simulink model "workingAUTOdec8"  (R2023b)
settings: Solver=FixedStepAuto  StartTime=0.0  StopTime=inf  RelTol=1e-3  EnableMultiTasking=on
libraries: vexarmcortexlib x17, vexcommonlib x4
settings Model: Creator=carol  LastModifiedBy=carol
settings SolverCC: AutoInsertRateTranBlk=on
settings DataIOCC: LimitDataPoints=on  SignalLoggingSaveFormat=ModelDataLogs  ReturnWorkspaceOutputs=off
settings OptimizationCC: ExpressionDepthLimit=2147483647  LifeSpan=Inf  MaxStackSize=64  EfficientTunableParamExpr=on
settings DebuggingCC: MergeDetectMultiDrivingBlocksExec=none  InheritedTsInSrcMsg=none  MultiTaskCondExecSysMsg=none  FcnCallInpInsideContextMsg=warning  StateNameClashWarn=warning  SFUnexpectedBacktrackingDiag=warning  SFNoUnconditionalDefaultTransitionDiag=warning  SFExecutionAtInitializationDiag=none  ArithmeticOperatorsInVariantConditions=warning
settings HardwareCC: ProdBitPerPointer=32  ProdBitPerSizeT=32  ProdBitPerPtrDiffT=32  ProdLargestAtomicInteger=Long  ProdLargestAtomicFloat=Double  ProdIntDivRoundTo=Undefined  ProdWordSize=32  ProdHWDeviceType=ARM Compatible->ARM Cortex
settings ModelReferenceCC: EnableRefExpFcnMdlSchedulingChecks=on  PropagateSignalLabelsOutOfModel=off
settings SFSimCC: MATLABDynamicMemAlloc=off  CustomCodeUndefinedFunction=UseInterfaceOnly
settings RTWCC: Description=Embedded Coder  SystemTargetFile=ert.tlc  HardwareBoard=ARM Cortex-based VEX Microcontroller  TemplateMakefile=ert_default_tmf  Toolchain=GNU Tools for VEX ARM Cortex
settings CodeAppCC: IgnoreCustomStorageClasses=off  CustomSymbolStrType=$N$R$M  StateflowObjectComments=on  InternalIdentifier=Classic
settings ERTTargetCC: CodeReplacementLibrary=GCC ARM Cortex-M3  MultiwordLength=2048  ConvertIfToSwitch=off  SuppressUnreachableDefaultCases=off

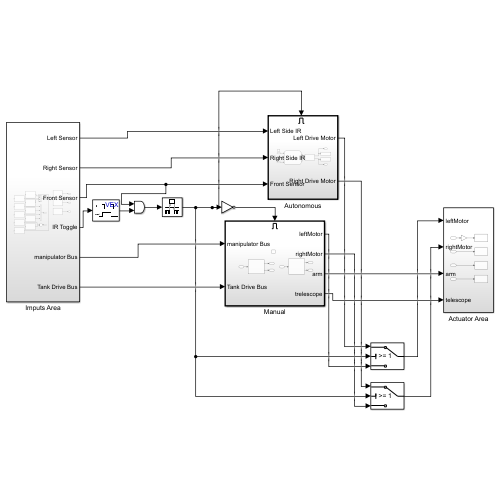
[thumbnail: Simulink's stored preview of the top-level diagram]
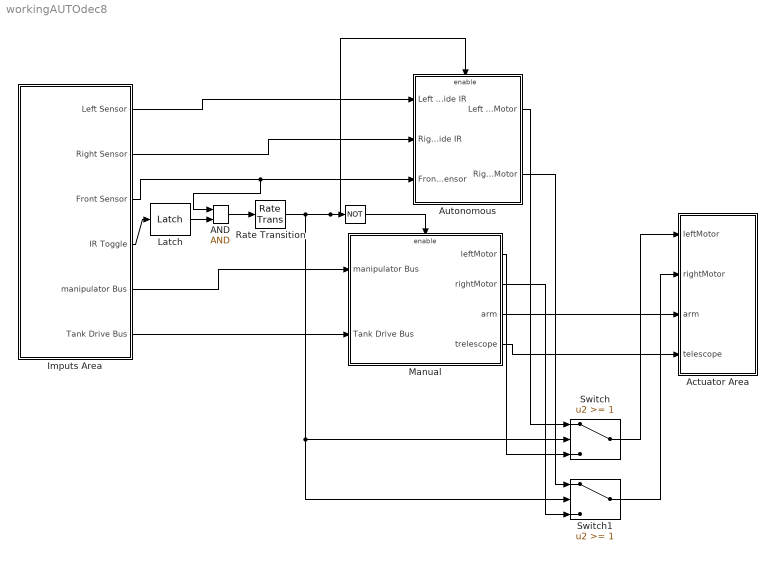
== system workingAUTOdec8 ==
  " " : Logic  Operator=NOT  IconShape=distinctive  AllPortsSameDT=off  OutDataTypeStr=boolean
  AND : Logic  IconShape=distinctive  AllPortsSameDT=off  OutDataTypeStr=boolean
  Actuator Area : Subsystem
  Autonomous : Subsystem  TreatAsAtomicUnit=on
  Imputs Area : Subsystem
  Latch : vexcommonlib/Latch  output0=off  BlockPlatform=vexarmcortex
  Manual : Subsystem  TreatAsAtomicUnit=on
  Rate Transition : RateTransition
  Switch : Switch  Threshold=1  SaturateOnIntegerOverflow=off  InputSameDT=off
  Switch1 : Switch  Threshold=1  SaturateOnIntegerOverflow=off  InputSameDT=off
  wires:
  Manual/3(arm) -> Actuator Area/3(arm)
  Manual/4(trelescope) -> Actuator Area/4(telescope)
  Switch1/1 -> Actuator Area/2(rightMotor)
  Switch/1 -> Actuator Area/1(leftMotor)
  Imputs Area/2(Right Sensor) -> Autonomous/2(Right Side IR)
  Imputs Area/3(Front Sensor) -> Autonomous/3(Front Sensor), AND/1
  Imputs Area/1(Left Sensor) -> Autonomous/1(Left Side IR)
  Imputs Area/5(manipulator Bus) -> Manual/1(manipulator Bus)
  Imputs Area/6(Tank Drive Bus) -> Manual/2(Tank Drive Bus)
  AND/1 -> Rate Transition/1
  Imputs Area/4(IR Toggle) -> Latch/1
  Latch/1 -> AND/2
  " "/1 -> Manual/Enable
  Autonomous/1(Left Drive Motor) -> Switch/1
  Manual/1(leftMotor) -> Switch/3
  Autonomous/2(Right Drive Motor) -> Switch1/1
  Manual/2(rightMotor) -> Switch1/3
  Rate Transition/1 -> Switch1/2, Switch/2, Autonomous/Enable, " "/1

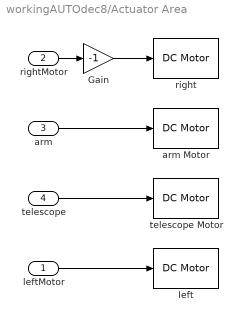
== system workingAUTOdec8/Actuator Area ==
  leftMotor : Inport
  rightMotor : Inport  Port=2
  arm : Inport  Port=3
  telescope : Inport  Port=4
  Gain : Gain  Gain=-1
  arm Motor : vexarmcortexlib/Actuators/DC Motor  motor=6  scaleFactor=1/13.5  SimulationOut=off
  left : vexarmcortexlib/Actuators/DC Motor  motor=9  scaleFactor=1/13.5  SimulationOut=off
  right : vexarmcortexlib/Actuators/DC Motor  motor=2  scaleFactor=1/13.5  SimulationOut=off
  telescope Motor : vexarmcortexlib/Actuators/DC Motor  motor=5  scaleFactor=1/13.5  SimulationOut=off
  wires:
  leftMotor/1 -> left/1
  arm/1 -> arm Motor/1
  rightMotor/1 -> Gain/1
  telescope/1 -> telescope Motor/1
  Gain/1 -> right/1

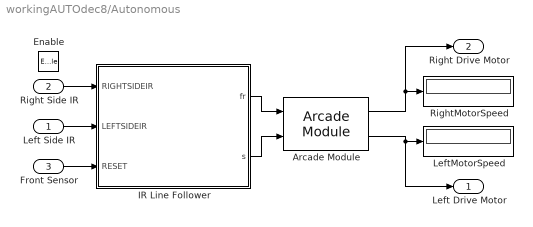
== system workingAUTOdec8/Autonomous ==
  Left Side IR : Inport
  Right Side IR : Inport  Port=2
  Front Sensor : Inport  Port=3
  Enable : EnablePort  StatesWhenEnabling=reset
  Arcade Module : vexcommonlib/Arcade Module  BlockPlatform=vexarmcortex
  IR Line Follower : Stateflow chart  TreatAsAtomicUnit=on
  LeftMotorSpeed : Display
  RightMotorSpeed : Display
  Left Drive Motor : Outport
  Right Drive Motor : Outport  Port=2
  wires:
  Arcade Module/2 -> LeftMotorSpeed/1, Left Drive Motor/1
  Arcade Module/1 -> Right Drive Motor/1, RightMotorSpeed/1
  Front Sensor/1 -> IR Line Follower/3(RESET)
  IR Line Follower/1(fr) -> Arcade Module/1
  IR Line Follower/2(s) -> Arcade Module/2
  Right Side IR/1 -> IR Line Follower/1(RIGHTSIDEIR)
  Left Side IR/1 -> IR Line Follower/2(LEFTSIDEIR)

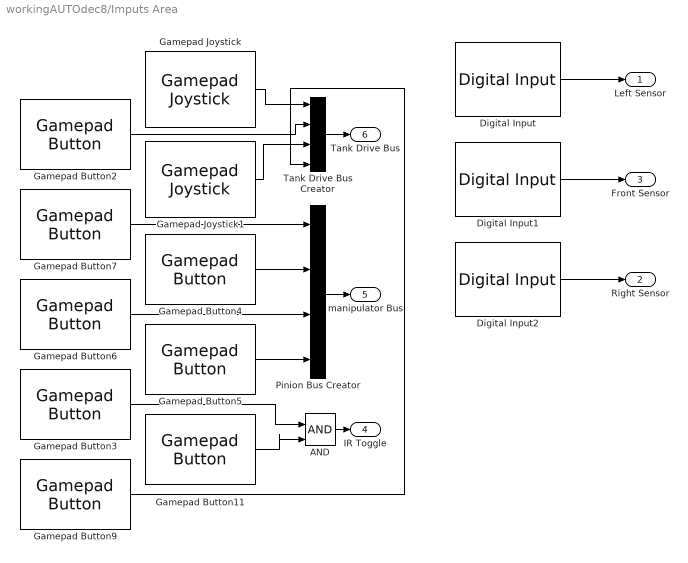
== system workingAUTOdec8/Imputs Area ==
  AND : Logic  IconShape=distinctive  AllPortsSameDT=off  OutDataTypeStr=boolean
  Digital Input : vexarmcortexlib/Sensors/Digital Input  inChan=10  SimulationIn=off  SampleTime=0.002
  Digital Input1 : vexarmcortexlib/Sensors/Digital Input  inChan=11  SimulationIn=off  SampleTime=0.002
  Digital Input2 : vexarmcortexlib/Sensors/Digital Input  inChan=12  SimulationIn=off  SampleTime=0.002
  Gamepad Button11 : vexarmcortexlib/Gamepad/Gamepad Button  joystick=1  chan=8  button56=Up  button78=Down  SimulationIn=on  SampleTime=0.02
  Gamepad Button2 : vexarmcortexlib/Gamepad/Gamepad Button  joystick=1  chan=7  button56=Up  button78=Right  SimulationIn=on  SampleTime=0.02
  Gamepad Button3 : vexarmcortexlib/Gamepad/Gamepad Button  joystick=1  chan=7  button56=Up  button78=Down  SimulationIn=on  SampleTime=0.02
  Gamepad Button4 : vexarmcortexlib/Gamepad/Gamepad Button  joystick=1  chan=5  button56=Down  button78=Down  SimulationIn=on  SampleTime=0.02
  Gamepad Button5 : vexarmcortexlib/Gamepad/Gamepad Button  joystick=1  chan=6  button56=Down  button78=Down  SimulationIn=on  SampleTime=0.02
  Gamepad Button6 : vexarmcortexlib/Gamepad/Gamepad Button  joystick=1  chan=6  button56=Up  button78=Down  SimulationIn=on  SampleTime=0.02
  Gamepad Button7 : vexarmcortexlib/Gamepad/Gamepad Button  joystick=1  chan=5  button56=Up  button78=Down  SimulationIn=on  SampleTime=0.02
  Gamepad Button9 : vexarmcortexlib/Gamepad/Gamepad Button  joystick=1  chan=8  button56=Up  button78=Up  SimulationIn=on  SampleTime=0.02
  Gamepad Joystick : vexarmcortexlib/Gamepad/Gamepad Joystick  joystick=1  chan=2  SimulationIn=on  SampleTime=0.02
  Gamepad Joystick1 : vexarmcortexlib/Gamepad/Gamepad Joystick  joystick=1  chan=3  SimulationIn=on  SampleTime=0.02
  Pinion Bus Creator : BusCreator  Inputs=4
  Tank Drive Bus Creator : BusCreator  Inputs=4
  Left Sensor : Outport
  Right Sensor : Outport  Port=2
  Front Sensor : Outport  Port=3
  IR Toggle : Outport  Port=4
  manipulator Bus : Outport  Port=5
  Tank Drive Bus : Outport  Port=6
  wires:
  Gamepad Joystick1/1 -> Tank Drive Bus Creator/3
  Gamepad Joystick/1 -> Tank Drive Bus Creator/1
  Gamepad Button7/1 -> Pinion Bus Creator/1
  Gamepad Button2/1 -> Tank Drive Bus Creator/2
  Gamepad Button6/1 -> Pinion Bus Creator/3
  Gamepad Button11/1 -> AND/2
  Gamepad Button5/1 -> Pinion Bus Creator/4
  Gamepad Button3/1 -> AND/1
  Gamepad Button4/1 -> Pinion Bus Creator/2
  Digital Input/1 -> Left Sensor/1
  Digital Input2/1 -> Right Sensor/1
  Digital Input1/1 -> Front Sensor/1
  Pinion Bus Creator/1 -> manipulator Bus/1
  Tank Drive Bus Creator/1 -> Tank Drive Bus/1
  AND/1 -> IR Toggle/1
  Gamepad Button9/1 -> Tank Drive Bus Creator/4

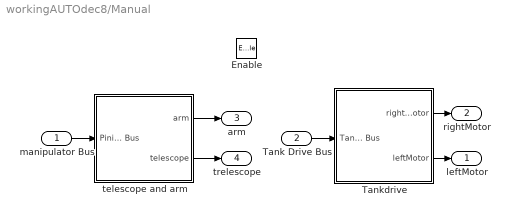
== system workingAUTOdec8/Manual ==
  manipulator Bus : Inport
  Tank Drive Bus : Inport  Port=2
  Enable : EnablePort
  Tankdrive : Subsystem
  telescope and arm : Subsystem
  leftMotor : Outport
  rightMotor : Outport  Port=2
  arm : Outport  Port=3
  trelescope : Outport  Port=4
  wires:
  telescope and arm/1(arm) -> arm/1
  telescope and arm/2(telescope) -> trelescope/1
  manipulator Bus/1 -> telescope and arm/1(Pinion Bus)
  Tank Drive Bus/1 -> Tankdrive/1(Tank Drive Bus)
  Tankdrive/1(rightMotor) -> rightMotor/1
  Tankdrive/2(leftMotor) -> leftMotor/1

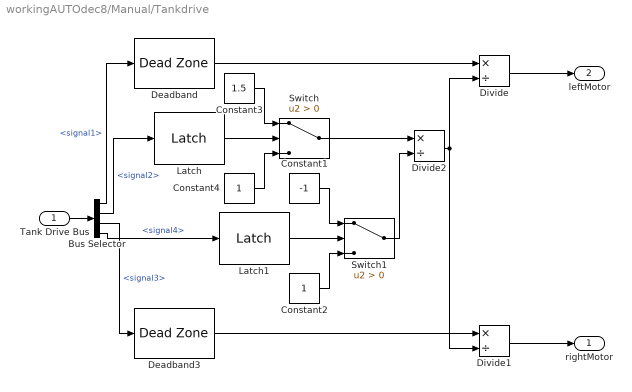
== system workingAUTOdec8/Manual/Tankdrive ==
  Tank Drive Bus : Inport
  Bus Selector : BusSelector  OutputSignals=signal1,signal2,signal3,signal4
  Constant1 : Constant  Value=-1
  Constant2 : Constant
  Constant3 : Constant  Value=1.5
  Constant4 : Constant
  Deadband : DeadZone  LowerValue=-9  UpperValue=9
  Deadband3 : DeadZone  LowerValue=-9  UpperValue=9
  Divide : Product  Inputs=*/
  Divide1 : Product  Inputs=*/
  Divide2 : Product  Inputs=*/
  Latch : vexcommonlib/Latch  output0=off  BlockPlatform=vexarmcortex
      settings: LibrarySourceBlock=vexarmcortexlib/Utilities/Latch
  Latch1 : vexcommonlib/Latch  output0=off  BlockPlatform=vexarmcortex
      settings: LibrarySourceBlock=vexarmcortexlib/Utilities/Latch
  Switch : Switch  Criteria=u2 > Threshold  SaturateOnIntegerOverflow=off  InputSameDT=off
  Switch1 : Switch  Criteria=u2 > Threshold  SaturateOnIntegerOverflow=off  InputSameDT=off
  rightMotor : Outport
  leftMotor : Outport  Port=2
  wires:
  Constant4/1 -> Switch/3
  Constant3/1 -> Switch/1
  Divide1/1 -> rightMotor/1
  Latch/1 -> Switch/2
  Deadband3/1 -> Divide1/1
  Deadband/1 -> Divide/1
  Divide/1 -> leftMotor/1
  Tank Drive Bus/1 -> Bus Selector/1
  Bus Selector/2 -> Latch/1  "<signal2>"
  Bus Selector/1 -> Deadband/1  "<signal1>"
  Bus Selector/3 -> Deadband3/1  "<signal3>"
  Latch1/1 -> Switch1/2
  Constant2/1 -> Switch1/3
  Constant1/1 -> Switch1/1
  Bus Selector/4 -> Latch1/1  "<signal4>"
  Switch/1 -> Divide2/1
  Switch1/1 -> Divide2/2
  Divide2/1 -> Divide1/2, Divide/2

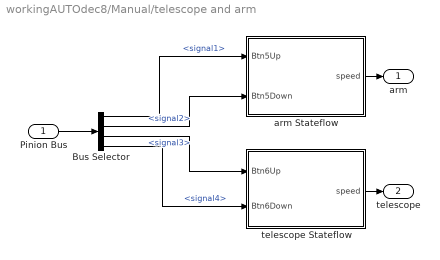
== system workingAUTOdec8/Manual/telescope and arm ==
  Pinion Bus : Inport
  Bus Selector : BusSelector  OutputSignals=signal1,signal2,signal3,signal4
  arm Stateflow : Stateflow chart  TreatAsAtomicUnit=on
  telescope Stateflow : Stateflow chart  TreatAsAtomicUnit=on
  arm : Outport
  telescope : Outport  Port=2
  wires:
  telescope Stateflow/1(speed) -> telescope/1
  arm Stateflow/1(speed) -> arm/1
  Bus Selector/1 -> arm Stateflow/1(Btn5Up)  "<signal1>"
  Pinion Bus/1 -> Bus Selector/1
  Bus Selector/2 -> arm Stateflow/2(Btn5Down)  "<signal2>"
  Bus Selector/3 -> telescope Stateflow/1(Btn6Up)  "<signal3>"
  Bus Selector/4 -> telescope Stateflow/2(Btn6Down)  "<signal4>"

== stateflow chart workingAUTOdec8/Manual/telescope and arm/arm Stateflow ==
  state rackIN
    entry:
    speed=-127;
  state STOPPED
    entry:
    speed=-20;
  state rackOUT
    entry:
    speed=127;
  (default) -> STOPPED
  STOPPED -> rackOUT [order 2] : [Btn5Down==0 && Btn5Up==1]
  STOPPED -> rackIN [order 1] : [Btn5Down==1 && Btn5Up==0]
  rackIN -> STOPPED [order 1] : [Btn5Down==0]
  rackOUT -> STOPPED [order 1] : [Btn5Up==0]
  rackIN -> STOPPED [order 2] : [Btn5Down==1 && Btn5Up==1]
  rackOUT -> STOPPED [order 2] : [Btn5Down==1 && Btn5Up==1]
  data: speed output; Btn5Up input; Btn5Down input

== stateflow chart workingAUTOdec8/Autonomous/IR Line Follower ==
  state STRAIGHT
    entry:
    fr = -75;
    s = 0;
  state GO_LEFT
    entry:
    fr =-30;
    s = 70;
  state GO_RIGHT
    entry:
    fr =-30;
    s = -70;
  state STOP
    entry:
    fr = 0;
    s = 0;
  (default) -> STRAIGHT
  GO_LEFT -> STRAIGHT [order 3] : [LEFTSIDEIR == 0 && RIGHTSIDEIR == 0]
  GO_RIGHT -> STRAIGHT [order 3] : [RIGHTSIDEIR == 0 && LEFTSIDEIR == 0]
  STRAIGHT -> GO_RIGHT [order 2] : [RIGHTSIDEIR == 0 && LEFTSIDEIR == 1]
  STRAIGHT -> GO_LEFT [order 1] : [LEFTSIDEIR == 0 && RIGHTSIDEIR ==1]
  STOP -> STRAIGHT [order 3] : [RIGHTSIDEIR == 0 && LEFTSIDEIR == 0 && RESET == 1]
  STRAIGHT -> STOP [order 3] : [RESET == 0]
  GO_LEFT -> GO_RIGHT [order 2] : [LEFTSIDEIR == 1 && RIGHTSIDEIR == 0]
  GO_RIGHT -> GO_LEFT [order 2] : [RIGHTSIDEIR == 1 && LEFTSIDEIR == 0]
  STOP -> GO_LEFT [order 2] : [RESET == 1 && LEFTSIDEIR == 0]
  GO_LEFT -> STOP [order 1] : [RESET == 0]
  STOP -> GO_RIGHT [order 1] : [RESET == 1 && RIGHTSIDEIR == 0]
  GO_RIGHT -> STOP [order 1] : [RESET == 0]
  data: RIGHTSIDEIR input; LEFTSIDEIR input; RESET input; fr output; s output

== stateflow chart workingAUTOdec8/Manual/telescope and arm/telescope Stateflow ==
  state rackIN
    entry:
    speed=-127;
  state STOPPED
    entry:
    speed=0;
  state rackOUT
    entry:
    speed=127;
  (default) -> STOPPED
  STOPPED -> rackOUT [order 2] : [Btn6Down==0 && Btn6Up==1]
  STOPPED -> rackIN [order 1] : [Btn6Down==1 && Btn6Up==0]
  rackIN -> STOPPED [order 1] : [Btn6Down==0]
  rackOUT -> STOPPED [order 1] : [Btn6Up==0]
  rackIN -> STOPPED [order 2] : [Btn6Down==1 && Btn6Up==1]
  rackOUT -> STOPPED [order 2] : [Btn6Down==1 && Btn6Up==1]
  data: Btn6Up input; Btn6Down input; speed output
